simulink model "privod"  (R2015a)
settings: Solver=ode45  StartTime=0.0  StopTime=10.0  RelTol=1e-3
settings Model: Creator=ANSYSVLAD  LastModifiedBy=ANSYSVLAD

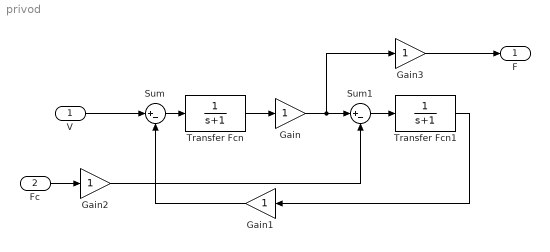
== system privod ==
  V : Inport
  Fc : Inport  Port=2
  Gain{,1..3} (4 alike) : Gain
  Sum : Sum  Inputs=|+-
  Sum1 : Sum  Inputs=|+-
  Transfer Fcn : TransferFcn  Denominator=[1 1]
  Transfer Fcn1 : TransferFcn  Denominator=[1 1]
  F : Outport
  wires:
  V/1 -> Sum/1
  Sum/1 -> Transfer Fcn/1
  Transfer Fcn/1 -> Gain/1
  Gain/1 -> Gain3/1, Sum1/1
  Sum1/1 -> Transfer Fcn1/1
  Gain1/1 -> Sum/2
  Transfer Fcn1/1 -> Gain1/1
  Fc/1 -> Gain2/1
  Gain2/1 -> Sum1/2
  Gain3/1 -> F/1
